simulink model "error_computation"  (R2017b)
settings: Solver=VariableStepAuto  StartTime=0.0  StopTime=10.0  RelTol=1e-3
undefined symbols (not defined in the file): I_i, path_info, tau_preview
settings Model: Creator=gimon  LastModifiedBy=gimon

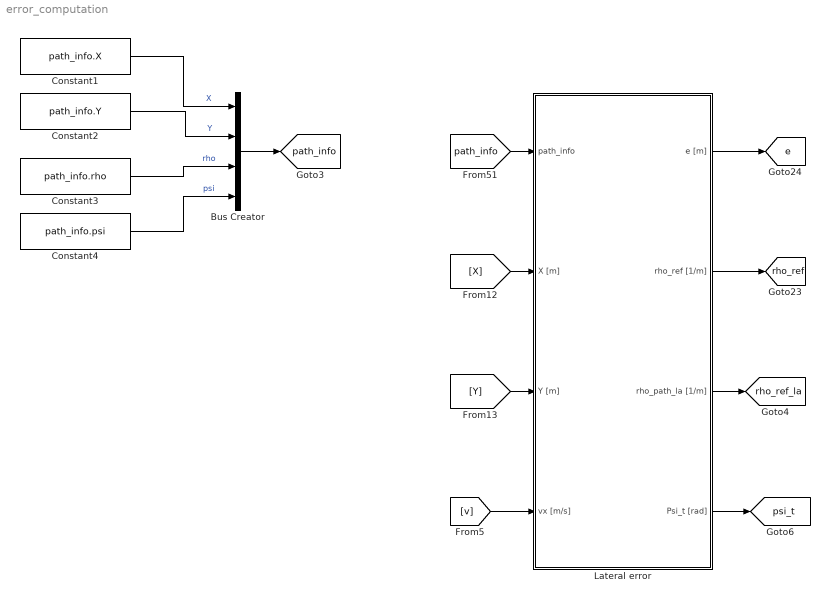
== system error_computation ==
  Bus Creator : BusCreator  Inputs=4
  Constant1 : Constant  Value=path_info.X
  Constant2 : Constant  Value=path_info.Y
  Constant3 : Constant  Value=path_info.rho
  Constant4 : Constant  Value=path_info.psi
  Lateral error : Subsystem
  tag scope: e=global, path_info=global, psi_t=global, rho_ref=global, rho_ref_la=global
  wires:
  Lateral error/4(Psi_t [rad]) -> [psi_t]
  [v] -> Lateral error/4(vx [m/s])
  Lateral error/2(rho_ref [1/m]) -> [rho_ref]
  Lateral error/1(e [m]) -> [e]
  Lateral error/3(rho_path_la [1/m]) -> [rho_ref_la]
  [Y] -> Lateral error/3(Y [m])
  [X] -> Lateral error/2(X [m])
  [path_info] -> Lateral error/1(path_info)
  Constant2/1 -> Bus Creator/2  "Y"
  Bus Creator/1 -> [path_info]
  Constant1/1 -> Bus Creator/1  "X"
  Constant3/1 -> Bus Creator/3  "rho"
  Constant4/1 -> Bus Creator/4  "psi"

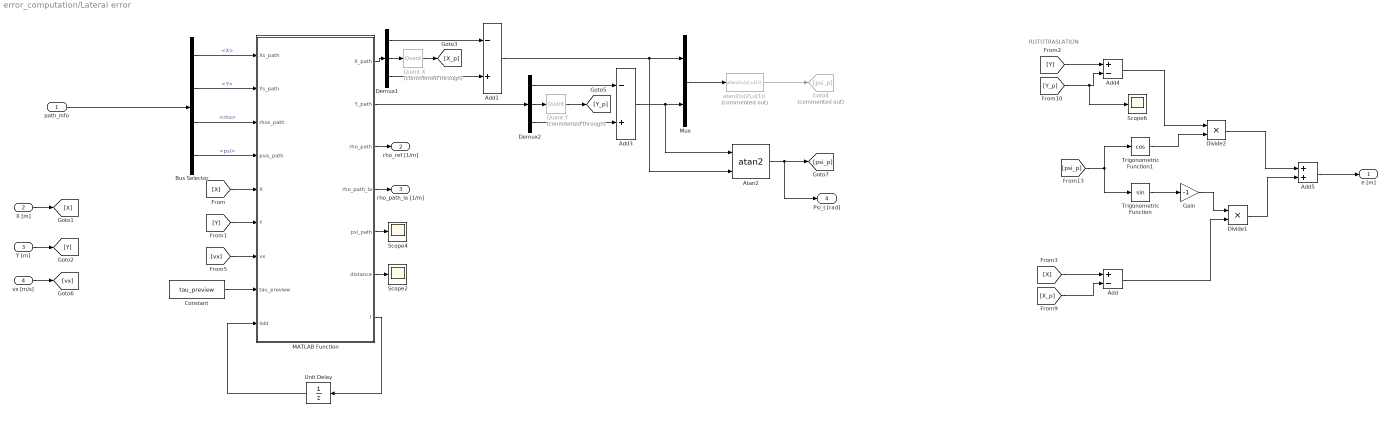
== system error_computation/Lateral error ==
  note: ROTOTRASLATION
  path_info : Inport
  X [m] : Inport  Port=2
  Y [m] : Inport  Port=3
  vx [m/s] : Inport  Port=4
  Add : Sum  Inputs=+-
  Add1 : Sum  Inputs=-+
  Add3 : Sum  Inputs=-+
  Add4 : Sum  Inputs=+-
  Add5 : Sum
  Atan2 : Trigonometry  Operator=atan2
  Bus Selector : BusSelector  OutputSignals=X,Y,rho,psi
  Constant : Constant  Value=tau_preview
  Demux1 : Demux  Outputs=3
  Demux2 : Demux  Outputs=3
  Divide1 : Product  Inputs=**
  Divide2 : Product  Inputs=**
  Gain : Gain  Gain=-1
  Goto4 : Goto  Commented=on  GotoTag=psi_p
  MATLAB Function : MATLAB Function  TreatAsAtomicUnit=on
  Mux : Mux  Inputs=2
  Quant X : Quantizer  Commented=through  QuantizationInterval=0.007
  Quant Y : Quantizer  Commented=through  QuantizationInterval=0.01
  Scope2 : Scope
  Scope4 : Scope
  Scope6 : Scope
  Trigonometric Function : Trigonometry
  Trigonometric Function1 : Trigonometry  Operator=cos
  Unit Delay : UnitDelay  InitialCondition=I_i  SampleTime=-1
  atan2(u(2),u(1)) : Fcn  Commented=on  Expr=atan2(u(2),u(1))
  e [m] : Outport
  rho_ref [1/m] : Outport  Port=2
  rho_path_la [1/m] : Outport  Port=3
  Psi_t [rad] : Outport  Port=4
  wires:
  Demux1/2 -> Quant X/1
  Demux1/3 -> Add1/2
  Add3/1 -> Atan2/1, Mux/2
  Demux2/2 -> Quant Y/1
  MATLAB Function/2(Y_path) -> Demux2/1
  Demux2/1 -> Add3/1
  Demux2/3 -> Add3/2
  MATLAB Function/3(rho_path) -> rho_ref [1/m]/1
  MATLAB Function/6(distance) -> Scope2/1
  MATLAB Function/1(X_path) -> Demux1/1
  Trigonometric Function1/1 -> Divide2/2
  Demux1/1 -> Add1/1
  MATLAB Function/7(I) -> Unit Delay/1
  [Y_p] -> Scope6/1, Add4/2
  Divide1/1 -> Add5/2
  Divide2/1 -> Add5/1
  [X_p] -> Add/2
  [psi_p] -> Trigonometric Function1/1, Trigonometric Function/1
  Trigonometric Function/1 -> Gain/1
  Add1/1 -> Atan2/2, Mux/1
  Unit Delay/1 -> MATLAB Function/9(Iold)
  Add/1 -> Divide1/2
  Add4/1 -> Divide2/1
  Gain/1 -> Divide1/1
  path_info/1 -> Bus Selector/1
  Bus Selector/1 -> MATLAB Function/1(Xs_path)  "<X>"
  Bus Selector/2 -> MATLAB Function/2(Ys_path)  "<Y>"
  Bus Selector/3 -> MATLAB Function/3(rhos_path)  "<rho>"
  Bus Selector/4 -> MATLAB Function/4(psis_path)  "<psi>"
  X [m]/1 -> [X]
  Y [m]/1 -> [Y]
  [X] -> MATLAB Function/5(X)
  [Y] -> MATLAB Function/6(Y)
  [Y] -> Add4/1
  [X] -> Add/1
  Quant X/1 -> [X_p]
  Quant Y/1 -> [Y_p]
  atan2(u(2),u(1))/1 -> Goto4/1
  MATLAB Function/5(psi_path) -> Scope4/1
  MATLAB Function/4(rho_path_la) -> rho_path_la [1/m]/1
  vx [m/s]/1 -> [vx]
  [vx] -> MATLAB Function/7(vx)
  Constant/1 -> MATLAB Function/8(tau_preview)
  Mux/1 -> atan2(u(2),u(1))/1
  Atan2/1 -> Psi_t [rad]/1, [psi_p]
  Add5/1 -> e [m]/1

== matlab function error_computation/Lateral error/MATLAB Function ==
  data: Xs_path input; Ys_path input; rhos_path input; psis_path input; X_path output; X input; Y input; vx input; tau_preview input; Y_path output; rho_path output; rho_path_la output; psi_path output; distance output; Iold input; I output
function [X_path,Y_path,rho_path,rho_path_la,psi_path,distance,I] = fcn(Xs_path,Ys_path,rhos_path,psis_path,X,Y,vx,tau_preview,Iold)
% ...
% returns coordinates, heading and distance of the nearest path point
% do not consider the car going backwards 

I_max=min(Iold+100,length(Xs_path));

Xs_path_tmp=Xs_path(Iold:I_max);
Ys_path_tmp=Ys_path(Iold:I_max);

[distance,Itmp]=min(sqrt((Xs_path_tmp-X).^2+(Ys_path_tmp-Y).^2));

I=Iold+Itmp-1;

X_path=Xs_path(I-1:I+1);
Y_path=Ys_path(I-1:I+1);
rho_path=rhos_path(I);
psi_path=psis_path(I);

% takes the future curvature
ds=0.1;
time_advance_indices=round(vx*tau_preview/ds);
rho_path_la=rhos_path(I+time_advance_indices);
